simulink model "sim1"  (R2015b)
settings: Solver=VariableStepAuto  StartTime=0.0  StopTime=20.0  RelTol=1e-3
settings Model: Creator=z  LastModifiedBy=z

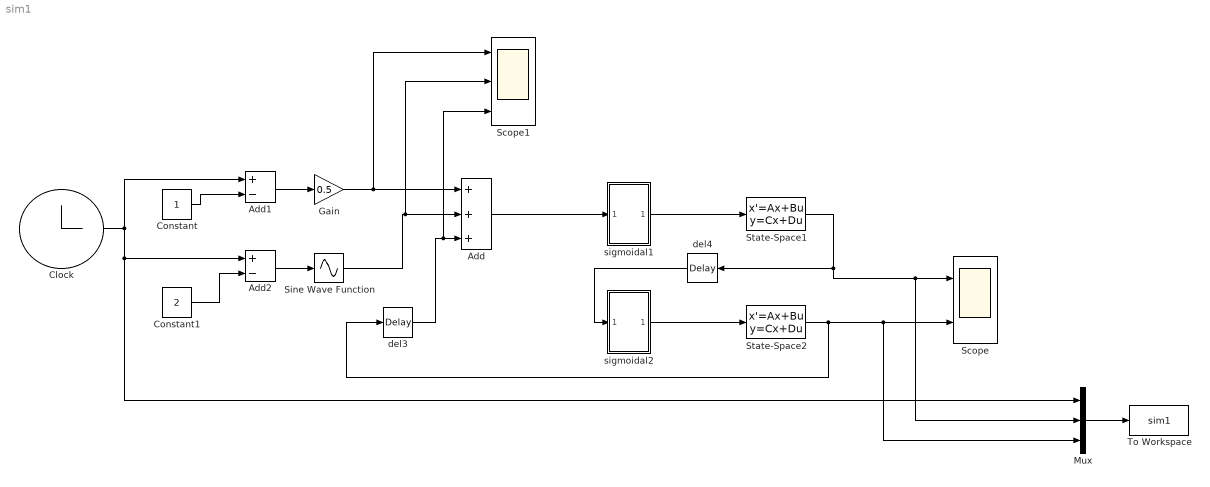
== system sim1 ==
  Add : Sum  Inputs=+++
  Add1 : Sum  Inputs=+-
  Add2 : Sum  Inputs=+-
  Clock : Clock
  Constant : Constant
  Constant1 : Constant  Value=2
  Gain : Gain  Gain=0.5
  Mux : Mux  Inputs=3
  Scope : Scope  NumInputPorts=2
  Scope1 : Scope  NumInputPorts=3
  Sine Wave Function : Sin  TimeSource=Use external signal  Amplitude=-4  SampleTime=0
  State-Space1 : StateSpace  A=-50  B=50  D=0  X0=.5  ContinuousStateAttributes='x'
  State-Space2 : StateSpace  A=-50  B=50  D=0  X0=0.5  ContinuousStateAttributes='y'
  To Workspace : ToWorkspace  VariableName=sim1  SampleTime=-1
  del3 : TransportDelay  DelayTime=6  InitialOutput=.5
  del4 : TransportDelay  DelayTime=5  InitialOutput=0.5
  sigmoidal1 : Subsystem
  sigmoidal2 : Subsystem
  wires:
  Add1/1 -> Gain/1
  Add2/1 -> Sine Wave Function/1
  Clock/1 -> Add1/1, Mux/1, Add2/1
  Gain/1 -> Scope1/1, Add/1
  Sine Wave Function/1 -> Scope1/2, Add/2
  State-Space1/1 -> del4/1, Mux/2, Scope/1
  Add/1 -> sigmoidal1/1(In1)
  sigmoidal1/1(Out1) -> State-Space1/1
  del3/1 -> Scope1/3, Add/3
  State-Space2/1 -> del3/1, Mux/3, Scope/2
  del4/1 -> sigmoidal2/1(In1)
  sigmoidal2/1(Out1) -> State-Space2/1
  Mux/1 -> To Workspace/1
  Constant/1 -> Add1/2
  Constant1/1 -> Add2/2

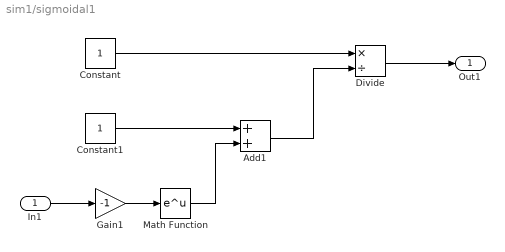
== system sim1/sigmoidal1 ==
  In1 : Inport
  Add1 : Sum
  Constant : Constant
  Constant1 : Constant
  Divide : Product  Inputs=*/
  Gain1 : Gain  Gain=-1
  Math Function : Math  SaturateOnIntegerOverflow=on
  Out1 : Outport
  wires:
  Constant1/1 -> Add1/1
  Gain1/1 -> Math Function/1
  Divide/1 -> Out1/1
  Constant/1 -> Divide/1
  In1/1 -> Gain1/1
  Add1/1 -> Divide/2
  Math Function/1 -> Add1/2

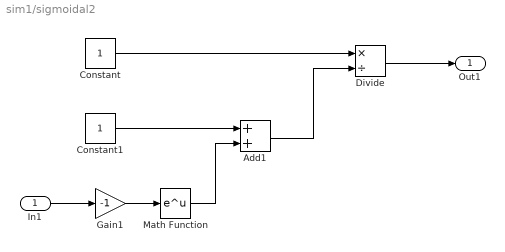
== system sim1/sigmoidal2 ==
  In1 : Inport
  Add1 : Sum
  Constant : Constant
  Constant1 : Constant
  Divide : Product  Inputs=*/
  Gain1 : Gain  Gain=-1
  Math Function : Math  SaturateOnIntegerOverflow=on
  Out1 : Outport
  wires:
  Constant1/1 -> Add1/1
  Gain1/1 -> Math Function/1
  Divide/1 -> Out1/1
  Constant/1 -> Divide/1
  In1/1 -> Gain1/1
  Add1/1 -> Divide/2
  Math Function/1 -> Add1/2
